simulink model "ads5296x4"  (R2018a)
settings: Solver=VariableStepAuto  StartTime=0.0  StopTime=10.0  RelTol=1e-3
libraries: xbsIndex_r4 x64
settings Model: Creator=qwerty40  LastModifiedBy=jackh
settings CodeAppCC: StateflowObjectComments=on

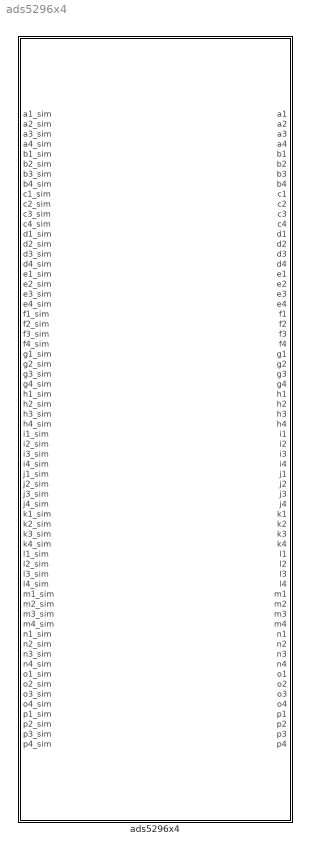
== system ads5296x4 ==
  ads5296x4 : Subsystem  Tag=xps:ads5296x4  mask(ADS5296x4){board_count=4}
      mask prompts: board_count "Number of quad-chip ADC Boards"
      mask help: 16-input ADC based on the TI ADS5296 chip.
      mask init:
      | % Only board_count is needed by init function
      | ads5296x4_init(gcb, ...
      |     'board_count', board_count);
      mask TypeOptions board_count: 1 | 2 | 3 | 4

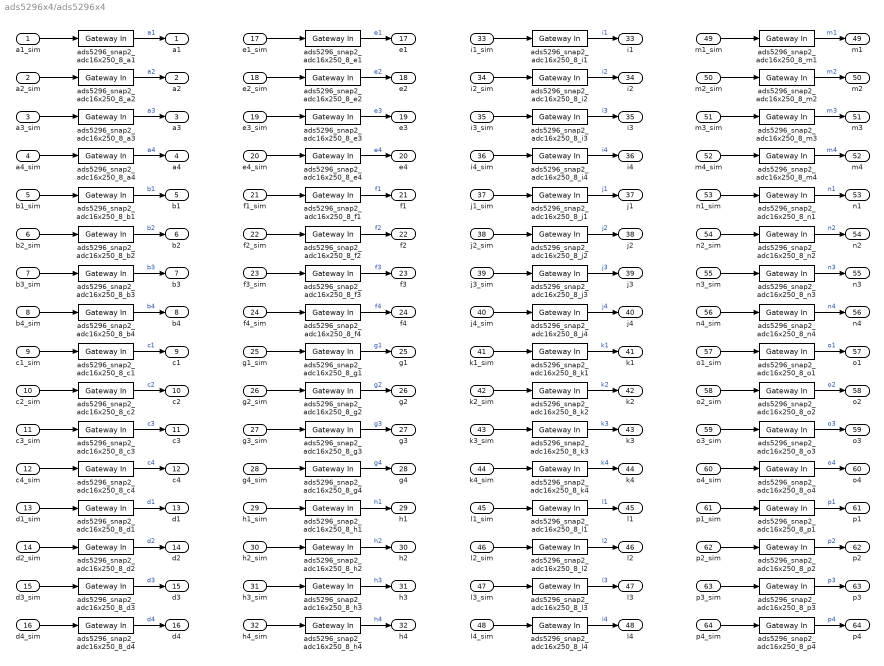
== system ads5296x4/ads5296x4 ==
  a1_sim : Inport
  a2_sim : Inport  Port=2
  a3_sim : Inport  Port=3
  a4_sim : Inport  Port=4
  b1_sim : Inport  Port=5
  b2_sim : Inport  Port=6
  b3_sim : Inport  Port=7
  b4_sim : Inport  Port=8
  c1_sim : Inport  Port=9
  c2_sim : Inport  Port=10
  c3_sim : Inport  Port=11
  c4_sim : Inport  Port=12
  d1_sim : Inport  Port=13
  d2_sim : Inport  Port=14
  d3_sim : Inport  Port=15
  d4_sim : Inport  Port=16
  e1_sim : Inport  Port=17
  e2_sim : Inport  Port=18
  e3_sim : Inport  Port=19
  e4_sim : Inport  Port=20
  f1_sim : Inport  Port=21
  f2_sim : Inport  Port=22
  f3_sim : Inport  Port=23
  f4_sim : Inport  Port=24
  g1_sim : Inport  Port=25
  g2_sim : Inport  Port=26
  g3_sim : Inport  Port=27
  g4_sim : Inport  Port=28
  h1_sim : Inport  Port=29
  h2_sim : Inport  Port=30
  h3_sim : Inport  Port=31
  h4_sim : Inport  Port=32
  i1_sim : Inport  Port=33
  i2_sim : Inport  Port=34
  i3_sim : Inport  Port=35
  i4_sim : Inport  Port=36
  j1_sim : Inport  Port=37
  j2_sim : Inport  Port=38
  j3_sim : Inport  Port=39
  j4_sim : Inport  Port=40
  k1_sim : Inport  Port=41
  k2_sim : Inport  Port=42
  k3_sim : Inport  Port=43
  k4_sim : Inport  Port=44
  l1_sim : Inport  Port=45
  l2_sim : Inport  Port=46
  l3_sim : Inport  Port=47
  l4_sim : Inport  Port=48
  m1_sim : Inport  Port=49
  m2_sim : Inport  Port=50
  m3_sim : Inport  Port=51
  m4_sim : Inport  Port=52
  n1_sim : Inport  Port=53
  n2_sim : Inport  Port=54
  n3_sim : Inport  Port=55
  n4_sim : Inport  Port=56
  o1_sim : Inport  Port=57
  o2_sim : Inport  Port=58
  o3_sim : Inport  Port=59
  o4_sim : Inport  Port=60
  p1_sim : Inport  Port=61
  p2_sim : Inport  Port=62
  p3_sim : Inport  Port=63
  p4_sim : Inport  Port=64
  ads5296_snap2_adc16x250_8_a{1..4} (4 alike) : xbsIndex_r4/Gateway In  gui_display_data_type=Fixed-point  arith_type="Signed  (2's comp)"  n_bits=10  bin_pt=9  preci_type=Single  exp_width=8  frac_width=24  rows=1  columns=1  quantization="Round  (unbiased: +/- Inf)"  overflow=Saturate  period=1  UseAsADC=off  ADCChannel='1'  interface=None  automatic_assignment=on  address_offset=hex2dec('00')  intf_name=''  intf_description=''  default_value=0  timing_constraint=None  locs_specified=off  LOCs={}  io_standard={}  inherit_from_input=off  hdl_port=on  dbl_ovrd=off  block_type=gatewayin
  ads5296_snap2_adc16x250_8_b{1..4} (4 alike) : xbsIndex_r4/Gateway In  gui_display_data_type=Fixed-point  arith_type="Signed  (2's comp)"  n_bits=10  bin_pt=9  preci_type=Single  exp_width=8  frac_width=24  rows=1  columns=1  quantization="Round  (unbiased: +/- Inf)"  overflow=Saturate  period=1  UseAsADC=off  ADCChannel='1'  interface=None  automatic_assignment=on  address_offset=hex2dec('00')  intf_name=''  intf_description=''  default_value=0  timing_constraint=None  locs_specified=off  LOCs={}  io_standard={}  inherit_from_input=off  hdl_port=on  dbl_ovrd=off  block_type=gatewayin
  ads5296_snap2_adc16x250_8_c{1..4} (4 alike) : xbsIndex_r4/Gateway In  gui_display_data_type=Fixed-point  arith_type="Signed  (2's comp)"  n_bits=10  bin_pt=9  preci_type=Single  exp_width=8  frac_width=24  rows=1  columns=1  quantization="Round  (unbiased: +/- Inf)"  overflow=Saturate  period=1  UseAsADC=off  ADCChannel='1'  interface=None  automatic_assignment=on  address_offset=hex2dec('00')  intf_name=''  intf_description=''  default_value=0  timing_constraint=None  locs_specified=off  LOCs={}  io_standard={}  inherit_from_input=off  hdl_port=on  dbl_ovrd=off  block_type=gatewayin
  ads5296_snap2_adc16x250_8_d{1..4} (4 alike) : xbsIndex_r4/Gateway In  gui_display_data_type=Fixed-point  arith_type="Signed  (2's comp)"  n_bits=10  bin_pt=9  preci_type=Single  exp_width=8  frac_width=24  rows=1  columns=1  quantization="Round  (unbiased: +/- Inf)"  overflow=Saturate  period=1  UseAsADC=off  ADCChannel='1'  interface=None  automatic_assignment=on  address_offset=hex2dec('00')  intf_name=''  intf_description=''  default_value=0  timing_constraint=None  locs_specified=off  LOCs={}  io_standard={}  inherit_from_input=off  hdl_port=on  dbl_ovrd=off  block_type=gatewayin
  ads5296_snap2_adc16x250_8_e{1..4} (4 alike) : xbsIndex_r4/Gateway In  gui_display_data_type=Fixed-point  arith_type="Signed  (2's comp)"  n_bits=10  bin_pt=9  preci_type=Single  exp_width=8  frac_width=24  rows=1  columns=1  quantization="Round  (unbiased: +/- Inf)"  overflow=Saturate  period=1  UseAsADC=off  ADCChannel='1'  interface=None  automatic_assignment=on  address_offset=hex2dec('00')  intf_name=''  intf_description=''  default_value=0  timing_constraint=None  locs_specified=off  LOCs={}  io_standard={}  inherit_from_input=off  hdl_port=on  dbl_ovrd=off  block_type=gatewayin
  ads5296_snap2_adc16x250_8_f{1..4} (4 alike) : xbsIndex_r4/Gateway In  gui_display_data_type=Fixed-point  arith_type="Signed  (2's comp)"  n_bits=10  bin_pt=9  preci_type=Single  exp_width=8  frac_width=24  rows=1  columns=1  quantization="Round  (unbiased: +/- Inf)"  overflow=Saturate  period=1  UseAsADC=off  ADCChannel='1'  interface=None  automatic_assignment=on  address_offset=hex2dec('00')  intf_name=''  intf_description=''  default_value=0  timing_constraint=None  locs_specified=off  LOCs={}  io_standard={}  inherit_from_input=off  hdl_port=on  dbl_ovrd=off  block_type=gatewayin
  ads5296_snap2_adc16x250_8_g{1..4} (4 alike) : xbsIndex_r4/Gateway In  gui_display_data_type=Fixed-point  arith_type="Signed  (2's comp)"  n_bits=10  bin_pt=9  preci_type=Single  exp_width=8  frac_width=24  rows=1  columns=1  quantization="Round  (unbiased: +/- Inf)"  overflow=Saturate  period=1  UseAsADC=off  ADCChannel='1'  interface=None  automatic_assignment=on  address_offset=hex2dec('00')  intf_name=''  intf_description=''  default_value=0  timing_constraint=None  locs_specified=off  LOCs={}  io_standard={}  inherit_from_input=off  hdl_port=on  dbl_ovrd=off  block_type=gatewayin
  ads5296_snap2_adc16x250_8_h{1..4} (4 alike) : xbsIndex_r4/Gateway In  gui_display_data_type=Fixed-point  arith_type="Signed  (2's comp)"  n_bits=10  bin_pt=9  preci_type=Single  exp_width=8  frac_width=24  rows=1  columns=1  quantization="Round  (unbiased: +/- Inf)"  overflow=Saturate  period=1  UseAsADC=off  ADCChannel='1'  interface=None  automatic_assignment=on  address_offset=hex2dec('00')  intf_name=''  intf_description=''  default_value=0  timing_constraint=None  locs_specified=off  LOCs={}  io_standard={}  inherit_from_input=off  hdl_port=on  dbl_ovrd=off  block_type=gatewayin
  ads5296_snap2_adc16x250_8_i{1..4} (4 alike) : xbsIndex_r4/Gateway In  gui_display_data_type=Fixed-point  arith_type="Signed  (2's comp)"  n_bits=10  bin_pt=9  preci_type=Single  exp_width=8  frac_width=24  rows=1  columns=1  quantization="Round  (unbiased: +/- Inf)"  overflow=Saturate  period=1  UseAsADC=off  ADCChannel='1'  interface=None  automatic_assignment=on  address_offset=hex2dec('00')  intf_name=''  intf_description=''  default_value=0  timing_constraint=None  locs_specified=off  LOCs={}  io_standard={}  inherit_from_input=off  hdl_port=on  dbl_ovrd=off  block_type=gatewayin
  ads5296_snap2_adc16x250_8_j{1..4} (4 alike) : xbsIndex_r4/Gateway In  gui_display_data_type=Fixed-point  arith_type="Signed  (2's comp)"  n_bits=10  bin_pt=9  preci_type=Single  exp_width=8  frac_width=24  rows=1  columns=1  quantization="Round  (unbiased: +/- Inf)"  overflow=Saturate  period=1  UseAsADC=off  ADCChannel='1'  interface=None  automatic_assignment=on  address_offset=hex2dec('00')  intf_name=''  intf_description=''  default_value=0  timing_constraint=None  locs_specified=off  LOCs={}  io_standard={}  inherit_from_input=off  hdl_port=on  dbl_ovrd=off  block_type=gatewayin
  ads5296_snap2_adc16x250_8_k{1..4} (4 alike) : xbsIndex_r4/Gateway In  gui_display_data_type=Fixed-point  arith_type="Signed  (2's comp)"  n_bits=10  bin_pt=9  preci_type=Single  exp_width=8  frac_width=24  rows=1  columns=1  quantization="Round  (unbiased: +/- Inf)"  overflow=Saturate  period=1  UseAsADC=off  ADCChannel='1'  interface=None  automatic_assignment=on  address_offset=hex2dec('00')  intf_name=''  intf_description=''  default_value=0  timing_constraint=None  locs_specified=off  LOCs={}  io_standard={}  inherit_from_input=off  hdl_port=on  dbl_ovrd=off  block_type=gatewayin
  ads5296_snap2_adc16x250_8_l{1..4} (4 alike) : xbsIndex_r4/Gateway In  gui_display_data_type=Fixed-point  arith_type="Signed  (2's comp)"  n_bits=10  bin_pt=9  preci_type=Single  exp_width=8  frac_width=24  rows=1  columns=1  quantization="Round  (unbiased: +/- Inf)"  overflow=Saturate  period=1  UseAsADC=off  ADCChannel='1'  interface=None  automatic_assignment=on  address_offset=hex2dec('00')  intf_name=''  intf_description=''  default_value=0  timing_constraint=None  locs_specified=off  LOCs={}  io_standard={}  inherit_from_input=off  hdl_port=on  dbl_ovrd=off  block_type=gatewayin
  ads5296_snap2_adc16x250_8_m{1..4} (4 alike) : xbsIndex_r4/Gateway In  gui_display_data_type=Fixed-point  arith_type="Signed  (2's comp)"  n_bits=10  bin_pt=9  preci_type=Single  exp_width=8  frac_width=24  rows=1  columns=1  quantization="Round  (unbiased: +/- Inf)"  overflow=Saturate  period=1  UseAsADC=off  ADCChannel='1'  interface=None  automatic_assignment=on  address_offset=hex2dec('00')  intf_name=''  intf_description=''  default_value=0  timing_constraint=None  locs_specified=off  LOCs={}  io_standard={}  inherit_from_input=off  hdl_port=on  dbl_ovrd=off  block_type=gatewayin
  ads5296_snap2_adc16x250_8_n{1..4} (4 alike) : xbsIndex_r4/Gateway In  gui_display_data_type=Fixed-point  arith_type="Signed  (2's comp)"  n_bits=10  bin_pt=9  preci_type=Single  exp_width=8  frac_width=24  rows=1  columns=1  quantization="Round  (unbiased: +/- Inf)"  overflow=Saturate  period=1  UseAsADC=off  ADCChannel='1'  interface=None  automatic_assignment=on  address_offset=hex2dec('00')  intf_name=''  intf_description=''  default_value=0  timing_constraint=None  locs_specified=off  LOCs={}  io_standard={}  inherit_from_input=off  hdl_port=on  dbl_ovrd=off  block_type=gatewayin
  ads5296_snap2_adc16x250_8_o{1..4} (4 alike) : xbsIndex_r4/Gateway In  gui_display_data_type=Fixed-point  arith_type="Signed  (2's comp)"  n_bits=10  bin_pt=9  preci_type=Single  exp_width=8  frac_width=24  rows=1  columns=1  quantization="Round  (unbiased: +/- Inf)"  overflow=Saturate  period=1  UseAsADC=off  ADCChannel='1'  interface=None  automatic_assignment=on  address_offset=hex2dec('00')  intf_name=''  intf_description=''  default_value=0  timing_constraint=None  locs_specified=off  LOCs={}  io_standard={}  inherit_from_input=off  hdl_port=on  dbl_ovrd=off  block_type=gatewayin
  ads5296_snap2_adc16x250_8_p{1..4} (4 alike) : xbsIndex_r4/Gateway In  gui_display_data_type=Fixed-point  arith_type="Signed  (2's comp)"  n_bits=10  bin_pt=9  preci_type=Single  exp_width=8  frac_width=24  rows=1  columns=1  quantization="Round  (unbiased: +/- Inf)"  overflow=Saturate  period=1  UseAsADC=off  ADCChannel='1'  interface=None  automatic_assignment=on  address_offset=hex2dec('00')  intf_name=''  intf_description=''  default_value=0  timing_constraint=None  locs_specified=off  LOCs={}  io_standard={}  inherit_from_input=off  hdl_port=on  dbl_ovrd=off  block_type=gatewayin
  a1 : Outport
  a2 : Outport  Port=2
  a3 : Outport  Port=3
  a4 : Outport  Port=4
  b1 : Outport  Port=5
  b2 : Outport  Port=6
  b3 : Outport  Port=7
  b4 : Outport  Port=8
  c1 : Outport  Port=9
  c2 : Outport  Port=10
  c3 : Outport  Port=11
  c4 : Outport  Port=12
  d1 : Outport  Port=13
  d2 : Outport  Port=14
  d3 : Outport  Port=15
  d4 : Outport  Port=16
  e1 : Outport  Port=17
  e2 : Outport  Port=18
  e3 : Outport  Port=19
  e4 : Outport  Port=20
  f1 : Outport  Port=21
  f2 : Outport  Port=22
  f3 : Outport  Port=23
  f4 : Outport  Port=24
  g1 : Outport  Port=25
  g2 : Outport  Port=26
  g3 : Outport  Port=27
  g4 : Outport  Port=28
  h1 : Outport  Port=29
  h2 : Outport  Port=30
  h3 : Outport  Port=31
  h4 : Outport  Port=32
  i1 : Outport  Port=33
  i2 : Outport  Port=34
  i3 : Outport  Port=35
  i4 : Outport  Port=36
  j1 : Outport  Port=37
  j2 : Outport  Port=38
  j3 : Outport  Port=39
  j4 : Outport  Port=40
  k1 : Outport  Port=41
  k2 : Outport  Port=42
  k3 : Outport  Port=43
  k4 : Outport  Port=44
  l1 : Outport  Port=45
  l2 : Outport  Port=46
  l3 : Outport  Port=47
  l4 : Outport  Port=48
  m1 : Outport  Port=49
  m2 : Outport  Port=50
  m3 : Outport  Port=51
  m4 : Outport  Port=52
  n1 : Outport  Port=53
  n2 : Outport  Port=54
  n3 : Outport  Port=55
  n4 : Outport  Port=56
  o1 : Outport  Port=57
  o2 : Outport  Port=58
  o3 : Outport  Port=59
  o4 : Outport  Port=60
  p1 : Outport  Port=61
  p2 : Outport  Port=62
  p3 : Outport  Port=63
  p4 : Outport  Port=64
  wires:
  a1_sim/1 -> ads5296_snap2_adc16x250_8_a1/1
  ads5296_snap2_adc16x250_8_a1/1 -> a1/1  "a1"
  a2_sim/1 -> ads5296_snap2_adc16x250_8_a2/1
  ads5296_snap2_adc16x250_8_a2/1 -> a2/1  "a2"
  a3_sim/1 -> ads5296_snap2_adc16x250_8_a3/1
  ads5296_snap2_adc16x250_8_a3/1 -> a3/1  "a3"
  a4_sim/1 -> ads5296_snap2_adc16x250_8_a4/1
  ads5296_snap2_adc16x250_8_a4/1 -> a4/1  "a4"
  b1_sim/1 -> ads5296_snap2_adc16x250_8_b1/1
  ads5296_snap2_adc16x250_8_b1/1 -> b1/1  "b1"
  b2_sim/1 -> ads5296_snap2_adc16x250_8_b2/1
  ads5296_snap2_adc16x250_8_b2/1 -> b2/1  "b2"
  b3_sim/1 -> ads5296_snap2_adc16x250_8_b3/1
  ads5296_snap2_adc16x250_8_b3/1 -> b3/1  "b3"
  b4_sim/1 -> ads5296_snap2_adc16x250_8_b4/1
  ads5296_snap2_adc16x250_8_b4/1 -> b4/1  "b4"
  c1_sim/1 -> ads5296_snap2_adc16x250_8_c1/1
  ads5296_snap2_adc16x250_8_c1/1 -> c1/1  "c1"
  c2_sim/1 -> ads5296_snap2_adc16x250_8_c2/1
  ads5296_snap2_adc16x250_8_c2/1 -> c2/1  "c2"
  c3_sim/1 -> ads5296_snap2_adc16x250_8_c3/1
  ads5296_snap2_adc16x250_8_c3/1 -> c3/1  "c3"
  c4_sim/1 -> ads5296_snap2_adc16x250_8_c4/1
  ads5296_snap2_adc16x250_8_c4/1 -> c4/1  "c4"
  d1_sim/1 -> ads5296_snap2_adc16x250_8_d1/1
  ads5296_snap2_adc16x250_8_d1/1 -> d1/1  "d1"
  d2_sim/1 -> ads5296_snap2_adc16x250_8_d2/1
  ads5296_snap2_adc16x250_8_d2/1 -> d2/1  "d2"
  d3_sim/1 -> ads5296_snap2_adc16x250_8_d3/1
  ads5296_snap2_adc16x250_8_d3/1 -> d3/1  "d3"
  d4_sim/1 -> ads5296_snap2_adc16x250_8_d4/1
  ads5296_snap2_adc16x250_8_d4/1 -> d4/1  "d4"
  e1_sim/1 -> ads5296_snap2_adc16x250_8_e1/1
  ads5296_snap2_adc16x250_8_e1/1 -> e1/1  "e1"
  e2_sim/1 -> ads5296_snap2_adc16x250_8_e2/1
  ads5296_snap2_adc16x250_8_e2/1 -> e2/1  "e2"
  e3_sim/1 -> ads5296_snap2_adc16x250_8_e3/1
  ads5296_snap2_adc16x250_8_e3/1 -> e3/1  "e3"
  e4_sim/1 -> ads5296_snap2_adc16x250_8_e4/1
  ads5296_snap2_adc16x250_8_e4/1 -> e4/1  "e4"
  f1_sim/1 -> ads5296_snap2_adc16x250_8_f1/1
  ads5296_snap2_adc16x250_8_f1/1 -> f1/1  "f1"
  f2_sim/1 -> ads5296_snap2_adc16x250_8_f2/1
  ads5296_snap2_adc16x250_8_f2/1 -> f2/1  "f2"
  f3_sim/1 -> ads5296_snap2_adc16x250_8_f3/1
  ads5296_snap2_adc16x250_8_f3/1 -> f3/1  "f3"
  f4_sim/1 -> ads5296_snap2_adc16x250_8_f4/1
  ads5296_snap2_adc16x250_8_f4/1 -> f4/1  "f4"
  g1_sim/1 -> ads5296_snap2_adc16x250_8_g1/1
  ads5296_snap2_adc16x250_8_g1/1 -> g1/1  "g1"
  g2_sim/1 -> ads5296_snap2_adc16x250_8_g2/1
  ads5296_snap2_adc16x250_8_g2/1 -> g2/1  "g2"
  g3_sim/1 -> ads5296_snap2_adc16x250_8_g3/1
  ads5296_snap2_adc16x250_8_g3/1 -> g3/1  "g3"
  g4_sim/1 -> ads5296_snap2_adc16x250_8_g4/1
  ads5296_snap2_adc16x250_8_g4/1 -> g4/1  "g4"
  h1_sim/1 -> ads5296_snap2_adc16x250_8_h1/1
  ads5296_snap2_adc16x250_8_h1/1 -> h1/1  "h1"
  h2_sim/1 -> ads5296_snap2_adc16x250_8_h2/1
  ads5296_snap2_adc16x250_8_h2/1 -> h2/1  "h2"
  h3_sim/1 -> ads5296_snap2_adc16x250_8_h3/1
  ads5296_snap2_adc16x250_8_h3/1 -> h3/1  "h3"
  h4_sim/1 -> ads5296_snap2_adc16x250_8_h4/1
  ads5296_snap2_adc16x250_8_h4/1 -> h4/1  "h4"
  i1_sim/1 -> ads5296_snap2_adc16x250_8_i1/1
  ads5296_snap2_adc16x250_8_i1/1 -> i1/1  "i1"
  i2_sim/1 -> ads5296_snap2_adc16x250_8_i2/1
  ads5296_snap2_adc16x250_8_i2/1 -> i2/1  "i2"
  i3_sim/1 -> ads5296_snap2_adc16x250_8_i3/1
  ads5296_snap2_adc16x250_8_i3/1 -> i3/1  "i3"
  i4_sim/1 -> ads5296_snap2_adc16x250_8_i4/1
  ads5296_snap2_adc16x250_8_i4/1 -> i4/1  "i4"
  j1_sim/1 -> ads5296_snap2_adc16x250_8_j1/1
  ads5296_snap2_adc16x250_8_j1/1 -> j1/1  "j1"
  j2_sim/1 -> ads5296_snap2_adc16x250_8_j2/1
  ads5296_snap2_adc16x250_8_j2/1 -> j2/1  "j2"
  j3_sim/1 -> ads5296_snap2_adc16x250_8_j3/1
  ads5296_snap2_adc16x250_8_j3/1 -> j3/1  "j3"
  j4_sim/1 -> ads5296_snap2_adc16x250_8_j4/1
  ads5296_snap2_adc16x250_8_j4/1 -> j4/1  "j4"
  k1_sim/1 -> ads5296_snap2_adc16x250_8_k1/1
  ads5296_snap2_adc16x250_8_k1/1 -> k1/1  "k1"
  k2_sim/1 -> ads5296_snap2_adc16x250_8_k2/1
  ads5296_snap2_adc16x250_8_k2/1 -> k2/1  "k2"
  k3_sim/1 -> ads5296_snap2_adc16x250_8_k3/1
  ads5296_snap2_adc16x250_8_k3/1 -> k3/1  "k3"
  k4_sim/1 -> ads5296_snap2_adc16x250_8_k4/1
  ads5296_snap2_adc16x250_8_k4/1 -> k4/1  "k4"
  l1_sim/1 -> ads5296_snap2_adc16x250_8_l1/1
  ads5296_snap2_adc16x250_8_l1/1 -> l1/1  "l1"
  l2_sim/1 -> ads5296_snap2_adc16x250_8_l2/1
  ads5296_snap2_adc16x250_8_l2/1 -> l2/1  "l2"
  l3_sim/1 -> ads5296_snap2_adc16x250_8_l3/1
  ads5296_snap2_adc16x250_8_l3/1 -> l3/1  "l3"
  l4_sim/1 -> ads5296_snap2_adc16x250_8_l4/1
  ads5296_snap2_adc16x250_8_l4/1 -> l4/1  "l4"
  m1_sim/1 -> ads5296_snap2_adc16x250_8_m1/1
  ads5296_snap2_adc16x250_8_m1/1 -> m1/1  "m1"
  m2_sim/1 -> ads5296_snap2_adc16x250_8_m2/1
  ads5296_snap2_adc16x250_8_m2/1 -> m2/1  "m2"
  m3_sim/1 -> ads5296_snap2_adc16x250_8_m3/1
  ads5296_snap2_adc16x250_8_m3/1 -> m3/1  "m3"
  m4_sim/1 -> ads5296_snap2_adc16x250_8_m4/1
  ads5296_snap2_adc16x250_8_m4/1 -> m4/1  "m4"
  n1_sim/1 -> ads5296_snap2_adc16x250_8_n1/1
  ads5296_snap2_adc16x250_8_n1/1 -> n1/1  "n1"
  n2_sim/1 -> ads5296_snap2_adc16x250_8_n2/1
  ads5296_snap2_adc16x250_8_n2/1 -> n2/1  "n2"
  n3_sim/1 -> ads5296_snap2_adc16x250_8_n3/1
  ads5296_snap2_adc16x250_8_n3/1 -> n3/1  "n3"
  n4_sim/1 -> ads5296_snap2_adc16x250_8_n4/1
  ads5296_snap2_adc16x250_8_n4/1 -> n4/1  "n4"
  o1_sim/1 -> ads5296_snap2_adc16x250_8_o1/1
  ads5296_snap2_adc16x250_8_o1/1 -> o1/1  "o1"
  o2_sim/1 -> ads5296_snap2_adc16x250_8_o2/1
  ads5296_snap2_adc16x250_8_o2/1 -> o2/1  "o2"
  o3_sim/1 -> ads5296_snap2_adc16x250_8_o3/1
  ads5296_snap2_adc16x250_8_o3/1 -> o3/1  "o3"
  o4_sim/1 -> ads5296_snap2_adc16x250_8_o4/1
  ads5296_snap2_adc16x250_8_o4/1 -> o4/1  "o4"
  p1_sim/1 -> ads5296_snap2_adc16x250_8_p1/1
  ads5296_snap2_adc16x250_8_p1/1 -> p1/1  "p1"
  p2_sim/1 -> ads5296_snap2_adc16x250_8_p2/1
  ads5296_snap2_adc16x250_8_p2/1 -> p2/1  "p2"
  p3_sim/1 -> ads5296_snap2_adc16x250_8_p3/1
  ads5296_snap2_adc16x250_8_p3/1 -> p3/1  "p3"
  p4_sim/1 -> ads5296_snap2_adc16x250_8_p4/1
  ads5296_snap2_adc16x250_8_p4/1 -> p4/1  "p4"
